simulink model "mpc_example_2016b"  (R2016b)
settings: Solver=FixedStepDiscrete  StartTime=0.0  StopTime=st  FixedStep=T  RelTol=1e-3
values from neighbouring files (symbols this model uses):
  A = [ 1 T ... (first row only)    [example.m]
  B = [ 0 ... (first row only)    [example.m]
  C = [ 1 0 ]    [example.m]
  D = 0    [example.m]
  g = 9.8    [example.m]
  m = 2.5    [example.m]
  r = 20    [example.m]
  x0 = [ 0.2 ... (first row only)    [example.m]
libraries: mpclib x1
settings Model: Creator=Elkman  LastModifiedBy=Elkman

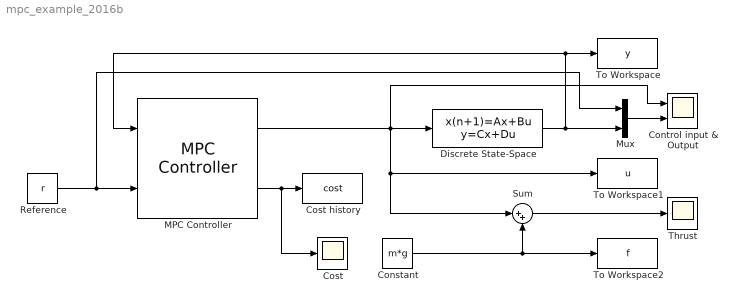
== system mpc_example_2016b ==
  Constant : Constant  Value=m*g
  Control input & Output : Scope  NumInputPorts=2
  Cost : Scope
  Cost history : ToWorkspace  VariableName=cost  SaveFormat=Timeseries  SampleTime=-1
  Discrete State-Space : DiscreteStateSpace  A=A  B=B  C=C  D=D  X0=x0  SampleTime=-1
  MPC Controller : mpclib/MPC Controller  SCDEnableBlockLinearizationSpecification=on  mpcobj=setmpc  is_multiple=0  enable_value=0  return_u0=off  ref_from_ws=off  ref_signal_name=[]  ref_preview=off  md_from_ws=off  md_signal_name=[]  md_preview=off  from_project=off  project_file=MPCtask.mat  md_inport=off  mv_inport=off  cost_outport=on  return_sequence=off  return_qpstatus=off  return_state=off  state_inport=off  lims_inport=off  ywt_inport=off  is_designfromscratch=0  uwt_inport=off  duwt_inport=off  rhoeps_inport=off  uref_inport=off  n_ts=0.2  n_mv=1  n_md=0  n_ud=0  n_mo=1  n_uo=0  BlockDataType=double  SampleTimeInherited=off  switch_inport=off
  Mux : Mux  Inputs=2
  Reference : Constant  Value=r
  Sum : Sum  Inputs=|++
  Thrust : Scope
  To Workspace : ToWorkspace  VariableName=y  SaveFormat=Timeseries  SampleTime=-1
  To Workspace1 : ToWorkspace  VariableName=u  SaveFormat=Timeseries  SampleTime=-1
  To Workspace2 : ToWorkspace  VariableName=f  SaveFormat=Timeseries  SampleTime=-1
  wires:
  Reference/1 -> Mux/1, MPC Controller/2
  Discrete State-Space/1 -> Mux/2, MPC Controller/1, To Workspace/1
  MPC Controller/1 -> Control input & Output/1, Discrete State-Space/1, Sum/1, To Workspace1/1
  Constant/1 -> To Workspace2/1, Sum/2
  Sum/1 -> Thrust/1
  Mux/1 -> Control input & Output/2
  MPC Controller/2 -> Cost/1, Cost history/1
